simulink model "F14_carrier_launch"  (R2025b)
settings: Solver=VariableStepAuto  StartTime=0.0  StopTime=6  MaxStep=0.01  RelTol=1e-3
values from neighbouring files (symbols this model uses):
  catapultcommand = [1 4 13]    [F_14_script.m]
  catapultforce = [5200000]    [F_14_script.m]
  Gp_den = [m c 0]    [F_14_script.m]
  Gp_num = [1]    [F_14_script.m]
  Gv_den = [m c]    [F_14_script.m]
  Gv_num = [1]    [F_14_script.m]
  K = 1/2*(density)*(lift_coefficient)*(wing_area)    (= 46.73375)    [F_14_script.m]
  throttle = [1 2]    [F_14_script.m]
  thrust_force = [500000]    [F_14_script.m]
settings Model: Creator=nuris  LastModifiedBy=nuris

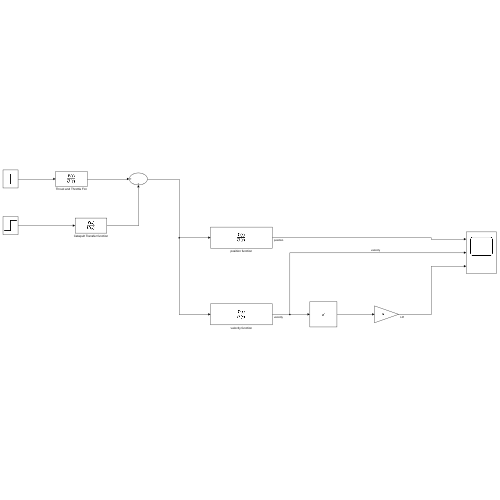
[thumbnail: Simulink's stored preview of the top-level diagram]
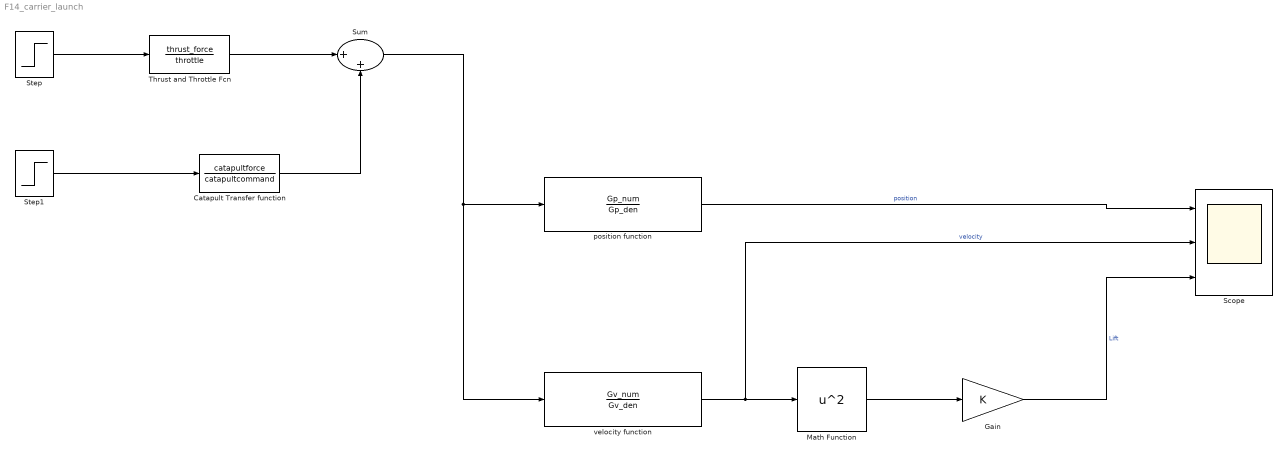
== system F14_carrier_launch ==
  Catapult Transfer function : TransferFcn  Numerator=catapultforce  Denominator=catapultcommand
  Gain : Gain  Gain=K
  Math Function : Math  Operator=square
  Scope : Scope  NumInputPorts=3
      settings: ActiveDisplayYMinimum=-65.882802117964772  ActiveDisplayYMaximum=592.945219061683
  Step : Step  Time=0  SampleTime=0
  Step1 : Step  Time=4  SampleTime=0
  Sum : Sum  Inputs=|++
  Thrust and Throttle Fcn : TransferFcn  Numerator=thrust_force  Denominator=throttle
  position function : TransferFcn  Numerator=Gp_num  Denominator=Gp_den
  velocity function : TransferFcn  Numerator=Gv_num  Denominator=Gv_den
  wires:
  Math Function/1 -> Gain/1
  velocity function/1 -> Scope/2, Math Function/1  "velocity"
  Step/1 -> Thrust and Throttle Fcn/1
  Thrust and Throttle Fcn/1 -> Sum/1
  Catapult Transfer function/1 -> Sum/2
  position function/1 -> Scope/1  "position"
  Gain/1 -> Scope/3  "Lift"
  Sum/1 -> position function/1, velocity function/1
  Step1/1 -> Catapult Transfer function/1
